simulink model "labTWOsecONE"  (R2023b)
settings: Solver=VariableStepAuto  StartTime=0.0  StopTime=10  RelTol=1e-3
settings Model: Creator=omarf  LastModifiedBy=omarf

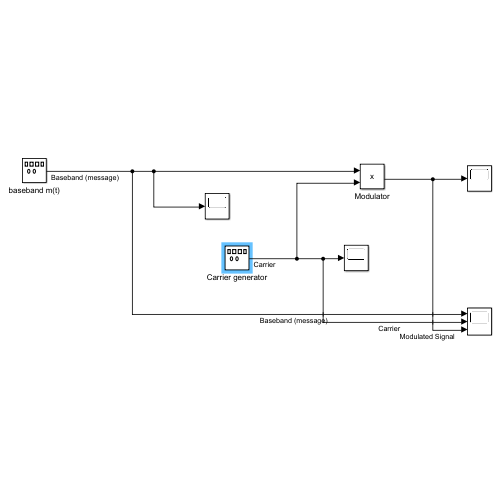
[thumbnail: Simulink's stored preview of the top-level diagram]
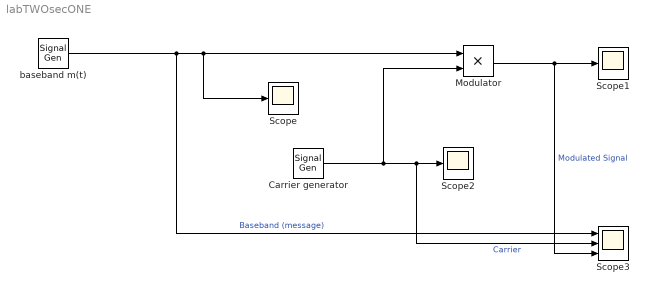
== system labTWOsecONE ==
  Carrier generator : SignalGenerator  Frequency=20000
  Modulator : Product
  Scope : Scope
  Scope1 : Scope
  Scope2 : Scope
  Scope3 : Scope  NumInputPorts=3
  baseband m(t) : SignalGenerator  Frequency=1000
  wires:
  Modulator/1 -> Scope3/3, Scope1/1  "Modulated Signal"
  baseband m(t)/1 -> Scope3/1, Scope/1, Modulator/1  "Baseband (message)"
  Carrier generator/1 -> Scope3/2, Scope2/1, Modulator/2  "Carrier"
